simulink model "firstSimulation"  (R2020b)
settings: Solver=VariableStepAuto  StartTime=0.0  StopTime=300.0  RelTol=1e-3
settings Model: Creator=sergio  LastModifiedBy=sergio

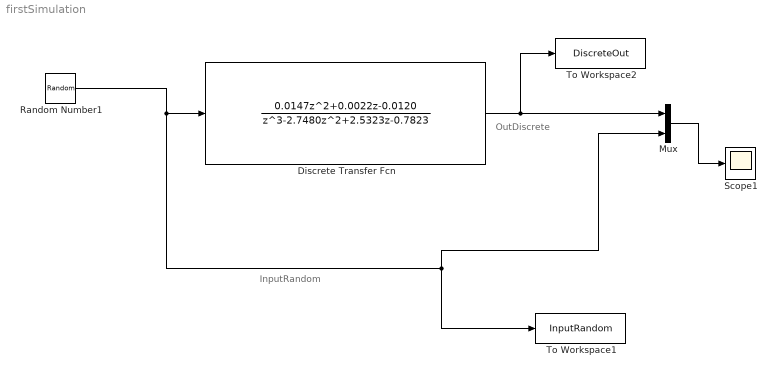
== system firstSimulation ==
  note: OutDiscrete
  note: InputRandom
  "Discrete Transfer Fcn " : DiscreteTransferFcn  Numerator=[0 0.0147 0.0022 -0.0120]  Denominator=[1.0000 -2.7480 2.5323 -0.7823]
  Mux : Mux  Inputs=2
  "Random Number1 " : RandomNumber  SampleTime=0.1
  "Scope1 " : Scope
  "To Workspace1 " : ToWorkspace  VariableName=InputRandom  SaveFormat=Timeseries  SampleTime=-1
  "To Workspace2 " : ToWorkspace  VariableName=DiscreteOut  SaveFormat=Timeseries  SampleTime=-1
  wires:
  "Random Number1 "/1 -> Mux/2, "To Workspace1 "/1, "Discrete Transfer Fcn "/1
  Mux/1 -> "Scope1 "/1
  "Discrete Transfer Fcn "/1 -> Mux/1, "To Workspace2 "/1
